simulink library "pathFollowingCtrlAoATurbCoef_VarElvAzu_cl"  (R2022a)
settings: Solver=VariableStepAuto  StartTime=0.0  StopTime=10.0  RelTol=1e-3
undefined symbols (not defined in the file or in its folder): env, FLIGHTCONTROLLER, fltCtrl, flwSpd, hiLvlCtrl, initializeBussesFromBlock, vhcl
libraries: pathFollowingCtrlAoATurbCoef_cl x2, pathFollowingCtrlAoATurbOpt_cl x1, courseFollowLookAhead_cl x1, ctrlAllocMatrix3CompCoef_cl x1, rotorTorqueCtrlDiscrete x1
settings Model: Creator=jbfine  LastModifiedBy=jbfine

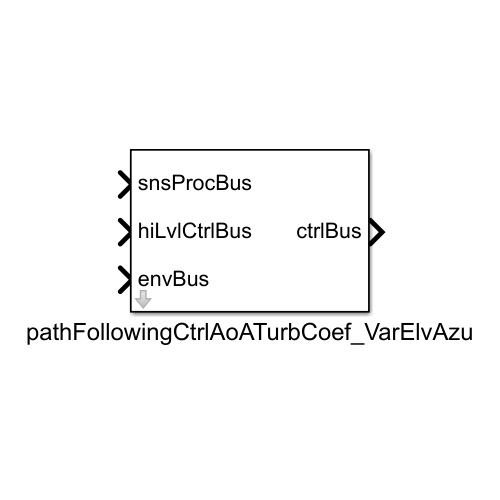
[thumbnail: Simulink's stored preview of the top-level diagram]
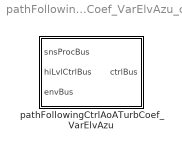
== system pathFollowingCtrlAoATurbCoef_VarElvAzu_cl ==
  pathFollowingCtrlAoATurbCoef_VarElvAzu : Subsystem  LoadFcn=initializeBussesFromBlock(gcb);  InitFcn=initializeBussesFromBlock(gcb);  VariantControl=strcmpi(FLIGHTCONTROLLER,'pathFollowingCtrlAoATurbCoef_varElvAzu')  mask{initPosForInitSStar=vhcl.initPosVecGnd.Value, fluidDensity=env.water.density.Value, pathCtrl=fltCtrl, aeroStruct=vhcl.struct('OCT.aeroSurf')}
      mask prompts: initPosForInitSStar "Initial Position"; fluidDensity "Fluid Density"; pathCtrl "Controller"; aeroStruct "Aerodynamic Structure"
      settings: PreSaveFcn=initializeBussesFromBlock(gcb);
      mask DialogControl Container3 Prompt: courseFollow Params
      mask DialogControl Container4 Prompt: setpointToOutput Params

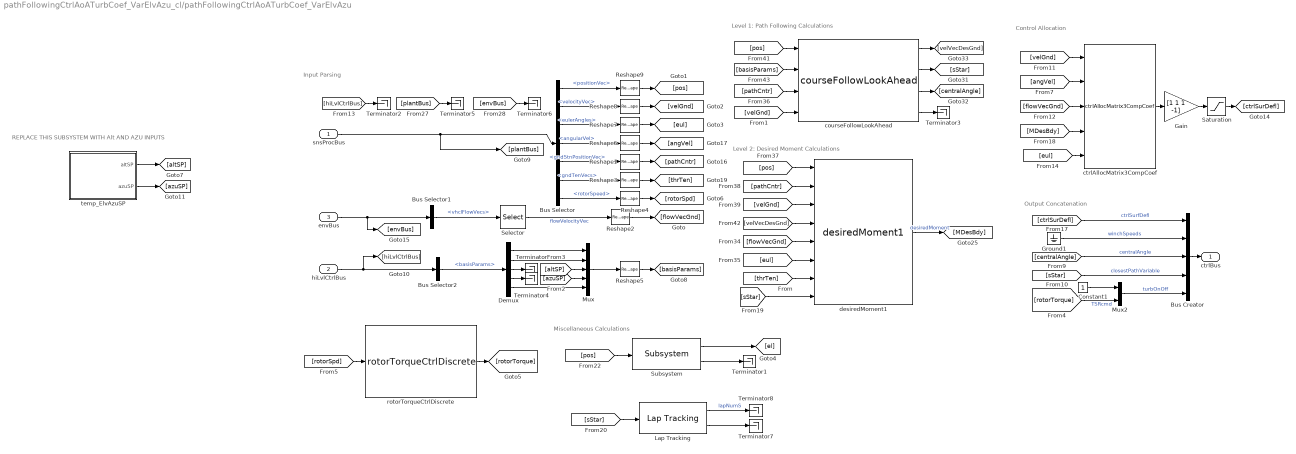
== system pathFollowingCtrlAoATurbCoef_VarElvAzu_cl/pathFollowingCtrlAoATurbCoef_VarElvAzu ==
  note: REPLACE THIS SUBSYSTEM WITH Alt AND AZU INPUTS
  note: Control Allocation
  note: Miscellaneous Calculations
  note: Level 2: Desired Moment Calculations
  note: Level 1: Path Following Calculations
  note: Output Concatenation
  note: Input Parsing
  snsProcBus : Inport  OutDataTypeStr=Bus: sensorsProcessingBus
  hiLvlCtrlBus : Inport  Port=2
  envBus : Inport  Port=3  OutDataTypeStr=Bus: envBus
  Bus Creator : BusCreator  Inputs=5
  Bus Selector : BusSelector  OutputSignals=positionVec,velocityVec,eulerAngles,angularVel,gndStnPositionVec,gndTenVecs,rotorSpeed
  Bus Selector1 : BusSelector  OutputSignals=vhclFlowVecs
  Bus Selector2 : BusSelector  OutputSignals=basisParams
  Constant1 : Constant
  Demux : Demux  Outputs=5
  Gain : Gain  Gain=[1 1 1 -1]
  Ground1 : Ground
  Lap Tracking : pathFollowingCtrlAoATurbOpt_cl/pathFollowingCtrlAoATurbOpt/Lap Tracking  SystemSampleTime=-1  VariantActivationTime=update diagram  Latency=0  AutoFrameSizeCalculation=off
  Mux : Mux  Inputs=5
  Mux2 : Mux  Inputs=2
  Reshape{1..9} (9 alike) : Reshape  OutputDimensionality=Column vector (2-D)
  Saturation : Saturate  UpperLimit=90  LowerLimit=-90
  Selector : Selector  NumberOfDimensions=2  InputPortWidth=3  IndexOptions=Select all,Index vector (dialog)  Indices=[1 3],5  OutputSizes=1,1
  Subsystem : pathFollowingCtrlAoATurbCoef_cl/pathFollowingCtrlAoATurbCoef/Subsystem  SystemSampleTime=-1  VariantActivationTime=update diagram  Latency=0  AutoFrameSizeCalculation=off
  Terminator{,1..8} (9 alike) : Terminator
  courseFollowLookAhead : courseFollowLookAhead_cl/courseFollowLookAhead  SystemSampleTime=-1  VariantActivationTime=update diagram  Latency=0  AutoFrameSizeCalculation=off
  ctrlAllocMatrix3CompCoef : ctrlAllocMatrix3CompCoef_cl/ctrlAllocMatrix3CompCoef  aeroStruct=vhcl.struct('OCT.aeroSurf')  fluidDensity=fluidDensity  arms=vhcl.struct('OCT.thrAttch')
  desiredMoment1 : pathFollowingCtrlAoATurbCoef_cl/pathFollowingCtrlAoATurbCoef/desiredMoment1  SystemSampleTime=-1  VariantActivationTime=update diagram  Latency=0  AutoFrameSizeCalculation=off
  rotorTorqueCtrlDiscrete : rotorTorqueCtrlDiscrete/rotorTorqueCtrlDiscrete  turb_struct=vhcl.struct('OCT.turb')  rho=rho
  temp_ElvAzuSP : Subsystem
  ctrlBus : Outport  OutDataTypeStr=Bus: fltCtrlBus  VectorParamsAs1DForOutWhenUnconnected=off
  wires:
  [angVel] -> ctrlAllocMatrix3CompCoef/2
  [velGnd] -> ctrlAllocMatrix3CompCoef/1
  Bus Selector/4 -> Reshape6/1  "<angularVel>"
  Reshape9/1 -> [pos]
  Reshape7/1 -> [eul]
  [ctrlSurDefl] -> Bus Creator/1  "ctrlSurfDefl"
  Bus Selector2/1 -> Demux/1  "<basisParams>"
  [pos] -> Subsystem/1
  [envBus] -> Terminator6/1
  [eul] -> desiredMoment1/6
  Reshape1/1 -> [pathCntr]
  [hiLvlCtrlBus] -> Terminator2/1
  [basisParams] -> courseFollowLookAhead/2
  [velGnd] -> desiredMoment1/3
  courseFollowLookAhead/1 -> [velVecDesGnd]
  courseFollowLookAhead/2 -> [sStar]
  Reshape4/1 -> [rotorSpd]
  [pos] -> courseFollowLookAhead/1
  [thrTen] -> desiredMoment1/7
  Gain/1 -> Saturation/1
  [velGnd] -> courseFollowLookAhead/4
  [pathCntr] -> desiredMoment1/2
  Reshape2/1 -> [flowVecGnd]
  [rotorTorque] -> Mux2/2  "TSRcmd"
  Constant1/1 -> Mux2/1
  Bus Selector/3 -> Reshape7/1  "<eulerAngles>"
  courseFollowLookAhead/4 -> Terminator3/1
  Bus Selector/6 -> Reshape3/1  "<gndTenVecs>"
  Reshape5/1 -> [basisParams]
  [flowVecGnd] -> ctrlAllocMatrix3CompCoef/3
  Subsystem/2 -> Terminator1/1
  [pathCntr] -> courseFollowLookAhead/3
  Bus Selector/2 -> Reshape8/1  "<velocityVec>"
  Reshape3/1 -> [thrTen]
  courseFollowLookAhead/3 -> [centralAngle]
  Bus Selector/1 -> Reshape9/1  "<positionVec>"
  Saturation/1 -> [ctrlSurDefl]
  [eul] -> ctrlAllocMatrix3CompCoef/5
  [plantBus] -> Terminator5/1
  Bus Selector/7 -> Reshape4/1  "<rotorSpeed>"
  Mux2/1 -> Bus Creator/5  "turbOnOff"
  snsProcBus/1 -> Bus Selector/1, [plantBus]
  Bus Selector/5 -> Reshape1/1  "<gndStnPositionVec>"
  [pos] -> desiredMoment1/1
  ctrlAllocMatrix3CompCoef/1 -> Gain/1
  hiLvlCtrlBus/1 -> Bus Selector2/1, [hiLvlCtrlBus]
  desiredMoment1/1 -> [MDesBdy]  "desiredMoment"
  Reshape8/1 -> [velGnd]
  Bus Creator/1 -> ctrlBus/1
  Subsystem/1 -> [el]
  Ground1/1 -> Bus Creator/2  "winchSpeeds"
  rotorTorqueCtrlDiscrete/1 -> [rotorTorque]
  [sStar] -> desiredMoment1/8
  Selector/1 -> Reshape2/1  "flowVelocityVec"
  [rotorSpd] -> rotorTorqueCtrlDiscrete/1
  [MDesBdy] -> ctrlAllocMatrix3CompCoef/4
  [flowVecGnd] -> desiredMoment1/5
  [sStar] -> Bus Creator/4  "closestPathVariable"
  [velVecDesGnd] -> desiredMoment1/4
  Reshape6/1 -> [angVel]
  [centralAngle] -> Bus Creator/3  "centralAngle"
  Bus Selector1/1 -> Selector/1  "<vhclFlowVecs>"
  envBus/1 -> Bus Selector1/1, [envBus]
  Mux/1 -> Reshape5/1
  Demux/1 -> Mux/1
  Demux/2 -> Mux/2
  Demux/5 -> Mux/5
  Demux/3 -> Terminator/1
  Demux/4 -> Terminator4/1
  [azuSP] -> Mux/4
  [altSP] -> Mux/3
  temp_ElvAzuSP/1(altSP) -> [altSP]
  temp_ElvAzuSP/2(azuSP) -> [azuSP]
  [sStar] -> Lap Tracking/1
  Lap Tracking/2 -> Terminator7/1
  Lap Tracking/1 -> Terminator8/1  "lapNumS"

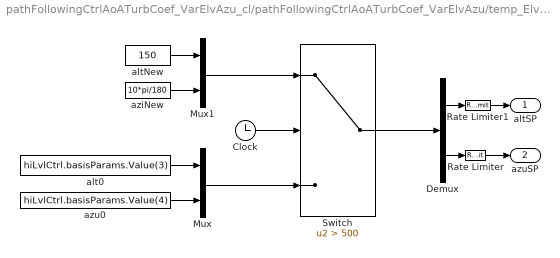
== system pathFollowingCtrlAoATurbCoef_VarElvAzu_cl/pathFollowingCtrlAoATurbCoef_VarElvAzu/temp_ElvAzuSP ==
  Clock : Clock
  Demux : Demux  Outputs=2
  Mux : Mux  Inputs=2
  Mux1 : Mux  Inputs=2
  Rate Limiter : RateLimiter  RisingSlewLimit=0.025*pi/180  FallingSlewLimit=-0.025*pi/180  SampleTimeMode=inherited
  Rate Limiter1 : RateLimiter  RisingSlewLimit=flwSpd/2  FallingSlewLimit=-flwSpd/2  SampleTimeMode=inherited
  Switch : Switch  Criteria=u2 > Threshold  Threshold=500  SaturateOnIntegerOverflow=off  InputSameDT=off
  alt0 : Constant  Value=hiLvlCtrl.basisParams.Value(3)
  altNew : Constant  Value=150
  aziNew : Constant  Value=10*pi/180  OutDataTypeStr=Inherit: Inherit via back propagation
  azu0 : Constant  Value=hiLvlCtrl.basisParams.Value(4)  OutDataTypeStr=Inherit: Inherit via back propagation
  altSP : Outport
  azuSP : Outport  Port=2
  wires:
  azu0/1 -> Mux/2
  alt0/1 -> Mux/1
  aziNew/1 -> Mux1/2
  altNew/1 -> Mux1/1
  Clock/1 -> Switch/2
  Mux1/1 -> Switch/1
  Mux/1 -> Switch/3
  Switch/1 -> Demux/1
  Demux/1 -> Rate Limiter1/1
  Demux/2 -> Rate Limiter/1
  Rate Limiter1/1 -> altSP/1
  Rate Limiter/1 -> azuSP/1
